simulink model "BLDCmotor_FOC_R2017b_fixdt_backup"  (R2017b)
settings: Solver=FixedStepDiscrete  StartTime=0  StopTime=0.5  FixedStep=Ts  MaxStep=1e-6  RelTol=1e-6  AbsTol=1e-6  EnableMultiTasking=on
PreLoadFcn:
  | addpath(pwd);
  | addpath(genpath('01_Libraries'));
  | addpath(genpath('02_Figures'));
  | addpath(genpath('03_CreateParamTable'));
InitFcn:
  | init_model;
values from neighbouring files (symbols this model uses):
  a_elecAngle = 60    [init_model.m]
  a_elecPeriod = 360    [init_model.m]
  a_phaAdvMax = 25    [init_model.m]
  b_angleMeasEna = 0    [init_model.m]
  b_cruiseCtrlEna = 0    [init_model.m]
  b_diagEna = 1    [init_model.m]
  b_fieldWeakEna = 0    [init_model.m]
  cf_currFilt = 0.12    [init_model.m]
  cf_idKi = 60 / (f_ctrl/3)    (= 0.01125)    [init_model.m]
  cf_idKp = 0.2    [init_model.m]
  cf_iqKi = 100 / (f_ctrl/3)    (= 0.01875)    [init_model.m]
  cf_iqKiLimProt = 60 / (f_ctrl/3)    (= 0.01125)    [init_model.m]
  cf_iqKp = 0.3    [init_model.m]
  cf_KbLimProt = 1000 / (f_ctrl/3)    (= 0.1875)    [init_model.m]
  cf_nKi = 20.4 / (f_ctrl/3)    (= 0.003825)    [init_model.m]
  cf_nKiLimProt = 20 / (f_ctrl/3)    (= 0.00375)    [init_model.m]
  cf_nKp = 1.18    [init_model.m]
  cf_speedCoef = round(f_ctrl * a_mechAngle * (pi/180) * (30/pi))    [init_model.m]
  CTRL_COM = 0    [init_model.m]
  CTRL_FOC = 2    [init_model.m]
  CTRL_SIN = 1    [init_model.m]
  dV_openRate = 1000 / (f_ctrl/3)    (= 0.1875)    [init_model.m]
  dz_cntTrnsDetHi = 40    [init_model.m]
  dz_cntTrnsDetLo = 20    [init_model.m]
  i_max = i_max * i_sca    (= 750)    [init_model.m]
  id_fieldWeakMax = 5 * i_sca    (= 250)    [init_model.m]
  iq_maxSca_M1 = sqrt(1 - iq_maxSca_XA.^2)    [init_model.m]
  n_commAcvLo = 15    [init_model.m]
  n_commDeacvHi = 30    [init_model.m]
  n_cruiseMotTgt = 0    [init_model.m]
  n_fieldWeakAuthHi = 400    [init_model.m]
  n_fieldWeakAuthLo = 300    [init_model.m]
  n_max = 1000    [init_model.m]
  n_polePairs = 15    [init_model.m]
  n_stdStillDet = 3    [init_model.m]
  OPEN_MODE = 0    [init_model.m]
  r_cos_M1 = cos((a_elecAngle_XA + 30)*(pi/180))    [init_model.m]
  r_errInpTgtThres = 600    [init_model.m]
  r_fieldWeakHi = 1000    [init_model.m]
  r_fieldWeakLo = 750    [init_model.m]
  r_sin3PhaA_M1 = sin3Arm + A*r_sinPhaA_M1    [init_model.m]
  r_sin3PhaB_M1 = sin3Arm + A*r_sinPhaB_M1    [init_model.m]
  r_sin3PhaC_M1 = sin3Arm + A*r_sinPhaC_M1    [init_model.m]
  r_sin_M1 = sin((a_elecAngle_XA + 30)*(pi/180))    [init_model.m]
  SPD_MODE = 2    [init_model.m]
  t_errDequal = 1.80 * f_ctrl/3    (= 9600)    [init_model.m]
  t_errQual = 0.24 * f_ctrl/3    (= 1280)    [init_model.m]
  TRQ_MODE = 3    [init_model.m]
  Ts = 5e-6    (= 5e-06)    [init_model.m]
  Ts_ctrl = 6e-5    (= 6e-05)    [init_model.m]
  Vd_max = 1000 - V_margin    (= 900)    [init_model.m]
  vec_hallToPos = [0 2 0 1 4 3 5 0]    [init_model.m]
  VLT_MODE = 1    [init_model.m]
  Vq_max_M1 = sqrt(Vd_max^2 - Vq_max_XA.^2)    [init_model.m]
  z_commutMap_M1 = [-1 -1  0  1  1  0 ... (first row only)    [init_model.m]
  z_ctrlModReq = VLT_MODE    (= 1)    [init_model.m]
  z_ctrlTypSel = CTRL_FOC    (= 2)    [init_model.m]
  z_maxCntRst = 2000    [init_model.m]
  z_selPhaCurMeasABC = 0    [init_model.m]
undefined symbols (not defined in the file or in its folder): DiscIntNeverNeededParam, sigbuilder_block
libraries: BLDC_controller_Lib x16, simulink x13, powerlib x6, pePwmGenerator x1
(part 3 of 4)

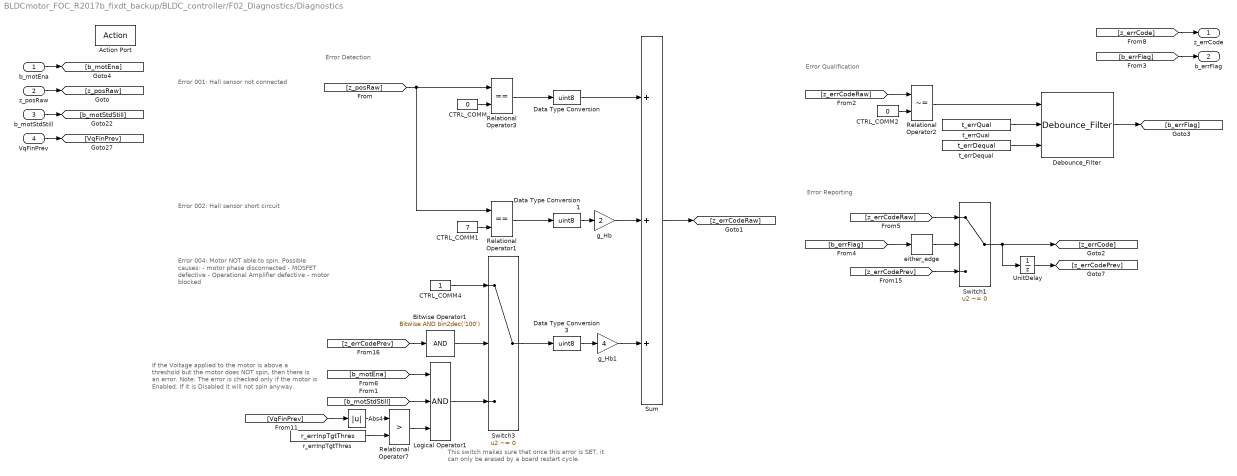
== system BLDCmotor_FOC_R2017b_fixdt_backup/BLDC_controller/F02_Diagnostics/Diagnostics ==
  note: Error 001: Hall sensor not connected
  note: Error 002: Hall sensor short circuit
  note: Error Qualification
  note: Error Detection
  note: Error Reporting
  note: Error 004: Motor NOT able to spin.
      |
      | Possible causes:
      | - motor phase disconnected
      | - MOSFET defective
      | - Operational Amplifier defective
      | - motor blocked
  note: This switch makes sure that once this error is SET, it can only be erased by a board restart cycle.
  note: If the Voltage applied to the motor is above a threshold but the motor does NOT spin, then there is an error.
      | Note: The error is checked only if the motor is Enabled. If it is Disabled it will not spin anyway.
  b_motEna : Inport
  z_posRaw : Inport  Port=2
  b_motStdStill : Inport  Port=3
  VqFinPrev : Inport  Port=4
  Action Port : ActionPort  ActionType=then
  Abs4 : Abs
  Bitwise Operator1 : simulink/Logic and Bit Operations/Bitwise Operator  logicop=AND  UseBitMask=on  BitMask=bin2dec('100')  BitMaskRealWorld=Stored Integer
  CTRL_COMM : Constant  Value=0  OutDataTypeStr=Inherit: Inherit via back propagation
  CTRL_COMM1 : Constant  Value=7  OutDataTypeStr=Inherit: Inherit via back propagation
  CTRL_COMM2 : Constant  Value=0  OutDataTypeStr=Inherit: Inherit via back propagation
  CTRL_COMM4 : Constant  OutDataTypeStr=Inherit: Inherit via back propagation
  Data Type Conversion : DataTypeConversion  OutDataTypeStr=uint8
  Data Type Conversion1 : DataTypeConversion  OutDataTypeStr=uint8
  Data Type Conversion3 : DataTypeConversion  OutDataTypeStr=uint8
  Debounce_Filter : BLDC_controller_Lib/Debounce_Filter
  Logical Operator1 : Logic  Inputs=3  AllPortsSameDT=off  OutDataTypeStr=boolean
  Relational Operator1 : RelationalOperator  Operator===  OutDataTypeStr=boolean  RndMeth=Simplest
  Relational Operator2 : RelationalOperator  Operator=~=  OutDataTypeStr=boolean  RndMeth=Simplest
  Relational Operator3 : RelationalOperator  Operator===  OutDataTypeStr=boolean  RndMeth=Simplest
  Relational Operator7 : RelationalOperator  Operator=>  OutDataTypeStr=boolean  RndMeth=Simplest
  Sum : Sum  Inputs=+++  RndMeth=Simplest  OutDataTypeStr=Inherit: Same as first input
  Switch1 : Switch  Criteria=u2 ~= 0  OutDataTypeStr=Inherit: Inherit via back propagation  RndMeth=Zero
  Switch3 : Switch  Criteria=u2 ~= 0  OutDataTypeStr=Inherit: Inherit via back propagation  RndMeth=Zero
  UnitDelay : UnitDelay  SampleTime=-1
      settings: AttributesFormatString=Ini=%<X0>
  either_edge : BLDC_controller_Lib/either_edge
  g_Hb : Gain  Gain=2  RndMeth=Simplest  OutDataTypeStr=Inherit: Same as input
  g_Hb1 : Gain  Gain=4  RndMeth=Simplest  OutDataTypeStr=Inherit: Same as input
  r_errInpTgtThres : Constant  Value=r_errInpTgtThres  OutDataTypeStr=Inherit: Inherit via back propagation
  t_errDequal : Constant  Value=t_errDequal  OutDataTypeStr=Inherit: Inherit via back propagation
  t_errQual : Constant  Value=t_errQual  OutDataTypeStr=Inherit: Inherit via back propagation
  "z_errCode " : Outport
  b_errFlag : Outport  Port=2
  wires:
  [z_errCode] -> "z_errCode "/1
  z_posRaw/1 -> [z_posRaw]
  t_errDequal/1 -> Debounce_Filter/3
  t_errQual/1 -> Debounce_Filter/2
  CTRL_COMM/1 -> Relational Operator3/2
  CTRL_COMM1/1 -> Relational Operator1/2
  [z_posRaw] -> Relational Operator1/1, Relational Operator3/1
  Relational Operator3/1 -> Data Type Conversion/1
  Sum/1 -> [z_errCodeRaw]
  Relational Operator2/1 -> Debounce_Filter/1
  [z_errCodeRaw] -> Relational Operator2/1
  CTRL_COMM2/1 -> Relational Operator2/2
  Debounce_Filter/1 -> [b_errFlag]
  either_edge/1 -> Switch1/2
  Switch1/1 -> [z_errCode], UnitDelay/1
  [b_errFlag] -> b_errFlag/1
  [b_errFlag] -> either_edge/1
  [z_errCodeRaw] -> Switch1/1
  g_Hb/1 -> Sum/2
  Relational Operator1/1 -> Data Type Conversion1/1
  Data Type Conversion/1 -> Sum/1
  Data Type Conversion1/1 -> g_Hb/1
  Switch3/1 -> Data Type Conversion3/1
  Data Type Conversion3/1 -> g_Hb1/1
  g_Hb1/1 -> Sum/3
  VqFinPrev/1 -> [VqFinPrev]
  b_motStdStill/1 -> [b_motStdStill]
  [VqFinPrev] -> Abs4/1
  Abs4/1 -> Relational Operator7/1
  r_errInpTgtThres/1 -> Relational Operator7/2
  UnitDelay/1 -> [z_errCodePrev]
  [z_errCodePrev] -> Switch1/3
  [z_errCodePrev] -> Bitwise Operator1/1
  Bitwise Operator1/1 -> Switch3/2
  CTRL_COMM4/1 -> Switch3/1
  Logical Operator1/1 -> Switch3/3
  b_motEna/1 -> [b_motEna]
  Relational Operator7/1 -> Logical Operator1/3
  [b_motEna] -> Logical Operator1/1
  [b_motStdStill] -> Logical Operator1/2

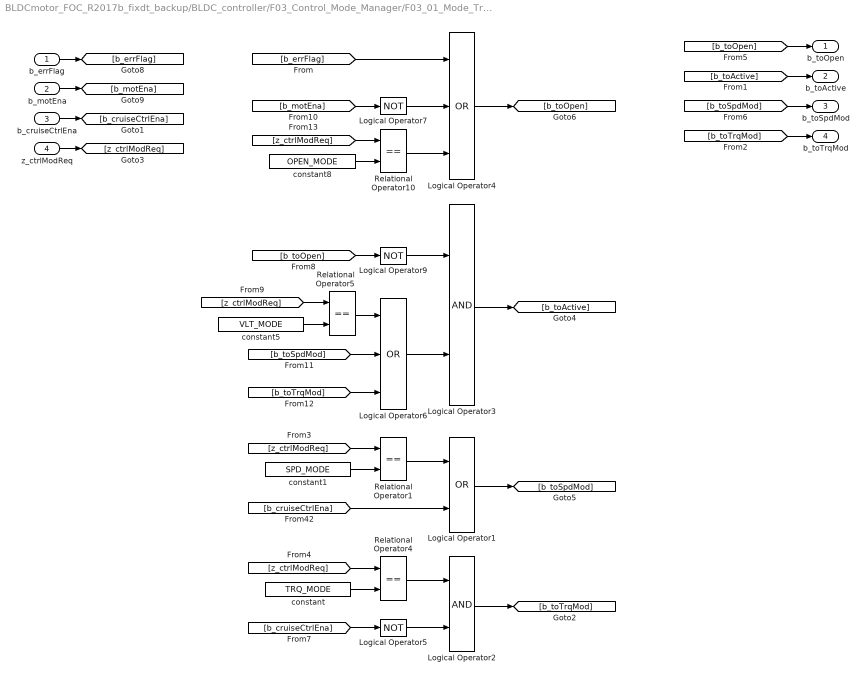
== system BLDCmotor_FOC_R2017b_fixdt_backup/BLDC_controller/F03_Control_Mode_Manager/F03_01_Mode_Transition_Calculation ==
  b_errFlag : Inport
  b_motEna : Inport  Port=2
  b_cruiseCtrlEna : Inport  Port=3
  z_ctrlModReq : Inport  Port=4
  Logical Operator1 : Logic  Operator=OR  AllPortsSameDT=off  OutDataTypeStr=boolean
  Logical Operator2 : Logic  AllPortsSameDT=off  OutDataTypeStr=boolean
  Logical Operator3 : Logic  AllPortsSameDT=off  OutDataTypeStr=boolean
  Logical Operator4 : Logic  Operator=OR  Inputs=3  AllPortsSameDT=off  OutDataTypeStr=boolean
  Logical Operator5 : Logic  Operator=NOT  AllPortsSameDT=off  OutDataTypeStr=boolean
  Logical Operator6 : Logic  Operator=OR  Inputs=3  AllPortsSameDT=off  OutDataTypeStr=boolean
  Logical Operator7 : Logic  Operator=NOT  AllPortsSameDT=off  OutDataTypeStr=boolean
  Logical Operator9 : Logic  Operator=NOT  AllPortsSameDT=off  OutDataTypeStr=boolean
  Relational Operator{1,4..5,10} (4 alike) : RelationalOperator  Operator===  OutDataTypeStr=boolean  RndMeth=Simplest
  constant : Constant  Value=TRQ_MODE  OutDataTypeStr=Inherit: Inherit via back propagation
  constant1 : Constant  Value=SPD_MODE  OutDataTypeStr=Inherit: Inherit via back propagation
  constant5 : Constant  Value=VLT_MODE  OutDataTypeStr=Inherit: Inherit via back propagation
  constant8 : Constant  Value=OPEN_MODE  OutDataTypeStr=Inherit: Inherit via back propagation
  b_toOpen : Outport  OutputWhenDisabled=reset  InitialOutput=0
  b_toActive : Outport  Port=2  OutputWhenDisabled=reset  InitialOutput=0
  b_toSpdMod : Outport  Port=3  OutputWhenDisabled=reset  InitialOutput=0
  b_toTrqMod : Outport  Port=4  OutputWhenDisabled=reset  InitialOutput=0
  wires:
  Logical Operator3/1 -> [b_toActive]
  [z_ctrlModReq] -> Relational Operator10/1
  constant5/1 -> Relational Operator5/2
  [z_ctrlModReq] -> Relational Operator4/1
  constant/1 -> Relational Operator4/2
  constant1/1 -> Relational Operator1/2
  [z_ctrlModReq] -> Relational Operator1/1
  Relational Operator5/1 -> Logical Operator6/1
  [z_ctrlModReq] -> Relational Operator5/1
  Logical Operator9/1 -> Logical Operator3/1
  Relational Operator10/1 -> Logical Operator4/3
  [b_motEna] -> Logical Operator7/1
  [b_toOpen] -> Logical Operator9/1
  Logical Operator4/1 -> [b_toOpen]
  constant8/1 -> Relational Operator10/2
  b_motEna/1 -> [b_motEna]
  z_ctrlModReq/1 -> [z_ctrlModReq]
  [b_toOpen] -> b_toOpen/1
  [b_toActive] -> b_toActive/1
  [b_toTrqMod] -> b_toTrqMod/1
  [b_toSpdMod] -> b_toSpdMod/1
  b_errFlag/1 -> [b_errFlag]
  [b_toSpdMod] -> Logical Operator6/2
  [b_toTrqMod] -> Logical Operator6/3
  Logical Operator6/1 -> Logical Operator3/2
  Relational Operator1/1 -> Logical Operator1/1
  Logical Operator1/1 -> [b_toSpdMod]
  [b_cruiseCtrlEna] -> Logical Operator1/2
  Relational Operator4/1 -> Logical Operator2/1
  Logical Operator2/1 -> [b_toTrqMod]
  [b_cruiseCtrlEna] -> Logical Operator5/1
  Logical Operator5/1 -> Logical Operator2/2
  Logical Operator7/1 -> Logical Operator4/2
  [b_errFlag] -> Logical Operator4/1
  b_cruiseCtrlEna/1 -> [b_cruiseCtrlEna]

== system BLDCmotor_FOC_R2017b_fixdt_backup/BLDC_controller/F03_Control_Mode_Manager/F03_03_Input_Target_Synthesis ==
  note: Input Scaling [-1000,1000] → [min,max]
  note: Final check if OPEN_MODE is requested
  z_ctrlTypSel : Inport
  z_ctrlModReq : Inport  Port=2
  z_ctrlMod : Inport  Port=3
  r_inpTgt : Inport  Port=4
  VqFinPrev : Inport  Port=5
  Default_Control_Type : Subsystem
  Default_Mode : Subsystem
  FOC_Control_Type : Subsystem
  If1 : If  IfExpression=u1 == CTRL_FOC
  If2 : If  IfExpression=u1 == OPEN_MODE
  Merge : Merge
  Merge1 : Merge
  Open_Mode : Subsystem
  Saturation : Saturate  UpperLimit=1000  LowerLimit=-1000
  r_inpTgtSca : Outport  OutputWhenDisabled=reset  InitialOutput=0
  wires:
  FOC_Control_Type/1(r_inpTgtScaFOC) -> Merge/1
  [r_inpTgt] -> FOC_Control_Type/1(r_inpTgt)
  [r_inpTgtSca] -> r_inpTgtSca/1
  If1/1 -> FOC_Control_Type/Action
  z_ctrlTypSel/1 -> [z_ctrlTypSel]
  [z_ctrlTypSel] -> If1/1
  Default_Control_Type/1(r_inpTgtScaDft) -> Merge/2
  [r_inpTgt] -> Default_Control_Type/1(r_inpTgt)
  r_inpTgt/1 -> Saturation/1
  Merge/1 -> [r_inpTgtScaRaw]
  If1/2 -> Default_Control_Type/Action
  [z_ctrlModReq] -> FOC_Control_Type/2(z_ctrlModReq)
  z_ctrlModReq/1 -> [z_ctrlModReq]
  z_ctrlMod/1 -> [z_ctrlMod]
  [z_ctrlMod] -> If2/1
  If2/1 -> Open_Mode/Action
  [VqFinPrev] -> Open_Mode/1(VqFinPrev)
  Open_Mode/1(r_inpTgtScaOpen) -> Merge1/1
  Default_Mode/1(r_inpTgtScaDft) -> Merge1/2
  Merge1/1 -> [r_inpTgtSca]
  [r_inpTgtScaRaw] -> Default_Mode/1(r_inpTgtScaRaw)
  If2/2 -> Default_Mode/Action
  VqFinPrev/1 -> [VqFinPrev]
  Saturation/1 -> [r_inpTgt]

== system BLDCmotor_FOC_R2017b_fixdt_backup/BLDC_controller/F04_Field_Weakening/Field_Weakening ==
  note: Calculate Blending Factor
  note: This blendig factor is a number between [0, 1]. It manages the Field weakening amount, ranging from 0 to a calibratable Max value.
  note: Field Weakening / Phase Advance
  z_ctrlTypSel : Inport
  r_inpTgt : Inport  Port=2
  n_motAbs : Inport  Port=3
  Action Port : ActionPort  ActionType=then
  Abs5 : Abs  OutDataTypeStr=Inherit: Inherit via back propagation  RndMeth=Zero
  CTRL_COMM2 : Constant  Value=CTRL_FOC  OutDataTypeStr=Inherit: Inherit via back propagation
  Divide1 : Product  Inputs=*/  OutDataTypeStr=fixdt(0,16,15)  RndMeth=Simplest
  Divide14 : Product  Inputs=*/  OutDataTypeStr=fixdt(0,16,15)  RndMeth=Simplest
  Divide2 : Product  Inputs=**  OutDataTypeStr=fixdt(0,16,15)  RndMeth=Simplest
  Divide3 : Product  Inputs=**  RndMeth=Simplest  OutDataTypeStr=Inherit: Same as first input
  Relational Operator1 : RelationalOperator  Operator===  OutDataTypeStr=boolean  RndMeth=Simplest
  Saturation Dynamic : simulink/Discontinuities/Saturation Dynamic  OutMin=[]  OutMax=[]  OutDataTypeStr=Inherit: Same as second input  OutDataType=fixdt(1, 16)  OutScaling=2^-10  DoSatur=off
  Saturation Dynamic1 : simulink/Discontinuities/Saturation Dynamic  OutMin=[]  OutMax=[]  OutDataTypeStr=Inherit: Same as second input  OutDataType=fixdt(1, 16)  OutScaling=2^-10  DoSatur=off
  Sum{1..4} (4 alike) : Sum  Inputs=+-  RndMeth=Simplest  OutDataTypeStr=Inherit: Same as first input
  Switch2 : Switch  Criteria=u2 ~= 0  OutDataTypeStr=Inherit: Inherit via back propagation  RndMeth=Zero
  a_phaAdvMax : Constant  Value=a_phaAdvMax  OutDataTypeStr=fixdt(1,16,4)
  id_fieldWeakMax : Constant  Value=id_fieldWeakMax  OutDataTypeStr=fixdt(1,16,4)
  n_fieldWeakAuthHi : Constant  Value=n_fieldWeakAuthHi  OutDataTypeStr=fixdt(1,16,4)
  n_fieldWeakAuthLo : Constant  Value=n_fieldWeakAuthLo  OutDataTypeStr=fixdt(1,16,4)
  r_fieldWeakHi : Constant  Value=r_fieldWeakHi  OutDataTypeStr=fixdt(1,16,4)
  r_fieldWeakLo : Constant  Value=r_fieldWeakLo  OutDataTypeStr=fixdt(1,16,4)
  "r_fieldWeak " : Outport
  wires:
  a_phaAdvMax/1 -> Switch2/3
  [r_fieldWeak] -> "r_fieldWeak "/1
  Switch2/1 -> Divide3/1
  n_fieldWeakAuthLo/1 -> Saturation Dynamic/3, Sum4/2, Sum2/2
  CTRL_COMM2/1 -> Relational Operator1/2
  Relational Operator1/1 -> Switch2/2
  [n_motAbs] -> Saturation Dynamic/2
  n_motAbs/1 -> [n_motAbs]
  Divide14/1 -> Divide2/1
  Saturation Dynamic/1 -> Sum4/1
  n_fieldWeakAuthHi/1 -> Saturation Dynamic/1, Sum2/1
  Divide1/1 -> Divide2/2
  Sum4/1 -> Divide1/1
  [r_blendFactor] -> Divide3/2
  Sum3/1 -> Divide14/2
  id_fieldWeakMax/1 -> Switch2/1
  [r_inpTgt] -> Abs5/1
  Saturation Dynamic1/1 -> Sum1/1
  Divide2/1 -> [r_blendFactor]
  Sum2/1 -> Divide1/2
  Abs5/1 -> Saturation Dynamic1/2
  z_ctrlTypSel/1 -> [z_ctrlTypSel]
  r_inpTgt/1 -> [r_inpTgt]
  r_fieldWeakHi/1 -> Saturation Dynamic1/1, Sum3/1
  r_fieldWeakLo/1 -> Saturation Dynamic1/3, Sum3/2, Sum1/2
  Divide3/1 -> [r_fieldWeak]
  Sum1/1 -> Divide14/1
  [z_ctrlTypSel] -> Relational Operator1/1

== system BLDCmotor_FOC_R2017b_fixdt_backup/BLDC_controller/F05_Field_Oriented_Control/Clarke_Transform ==
  i_phaAB : Inport
  i_phaBC : Inport  Port=2
  Clarke_PhasesAB : Subsystem
  Clarke_PhasesAC : Subsystem
  Clarke_PhasesBC : Subsystem
  If1 : If  IfExpression=u1 == 0  ElseIfExpressions=u1 == 1
  Merge1 : Merge  Inputs=3
  Merge2 : Merge  Inputs=3
  z_selPhaCurMeasABC : Constant  Value=z_selPhaCurMeasABC  OutDataTypeStr=uint8
  i_alpha : Outport
  i_beta : Outport  Port=2
  wires:
  Clarke_PhasesBC/1(i_alphaBC) -> [i_alphaBC]
  [i_betaBC] -> Merge1/2
  [i_betaAB] -> Merge1/1
  i_phaAB/1 -> [i_phaAB]
  [i_phaBC] -> Clarke_PhasesBC/2(i_phaC)
  [i_phaAB] -> Clarke_PhasesBC/1(i_phaB)
  Clarke_PhasesAB/1(i_alphaAB) -> [i_alphaAB]
  [i_alphaAB] -> Merge2/1
  If1/1 -> Clarke_PhasesAB/Action
  z_selPhaCurMeasABC/1 -> If1/1
  [i_alphaBC] -> Merge2/2
  [i_beta] -> i_beta/1
  Clarke_PhasesAB/2(i_betaAB) -> [i_betaAB]
  i_phaBC/1 -> [i_phaBC]
  [i_phaBC] -> Clarke_PhasesAB/2(i_phaB)
  Merge1/1 -> [i_beta]
  Merge2/1 -> [i_alpha]
  [i_phaAB] -> Clarke_PhasesAB/1(i_phaA)
  [i_alpha] -> i_alpha/1
  Clarke_PhasesBC/2(i_betaBC) -> [i_betaBC]
  If1/2 -> Clarke_PhasesBC/Action
  If1/3 -> Clarke_PhasesAC/Action
  [i_phaAB] -> Clarke_PhasesAC/1(i_phaA)
  [i_phaBC] -> Clarke_PhasesAC/2(i_phaC)
  Clarke_PhasesAC/2(i_betaAC) -> [i_betaAC]
  Clarke_PhasesAC/1(i_alphaAC) -> [i_alphaAC]
  [i_alphaAC] -> Merge2/3
  [i_betaAC] -> Merge1/3

== system BLDCmotor_FOC_R2017b_fixdt_backup/BLDC_controller/F05_Field_Oriented_Control/Current_Filtering ==
  iq_raw : Inport
  id_raw : Inport  Port=2
  Action Port : ActionPort  InitializeStates=reset  ActionType=then
  Abs5 : Abs  OutDataTypeStr=Inherit: Inherit via back propagation  RndMeth=Zero
  Demux1 : Demux  Outputs=2
  Low_Pass_Filter : BLDC_controller_Lib/Low_Pass_Filter  SystemSampleTime=-1
  Mux2 : Mux  Inputs=2
  cf_currFilt : Constant  Value=cf_currFilt  OutDataTypeStr=fixdt(0,16,16)
  iq : Outport  OutputWhenDisabled=reset  InitialOutput=0
  iqAbs : Outport  Port=2  OutputWhenDisabled=reset  InitialOutput=0
  id : Outport  Port=3  OutputWhenDisabled=reset  InitialOutput=0
  wires:
  Mux2/1 -> Low_Pass_Filter/1
  Demux1/2 -> [id]
  cf_currFilt/1 -> Low_Pass_Filter/2
  id_raw/1 -> [id_raw]
  [iq] -> Abs5/1, iq/1
  [id] -> id/1
  iq_raw/1 -> [iq_raw]
  Demux1/1 -> [iq]
  Low_Pass_Filter/1 -> Demux1/1
  [iq_raw] -> Mux2/1
  [id_raw] -> Mux2/2
  Abs5/1 -> iqAbs/1

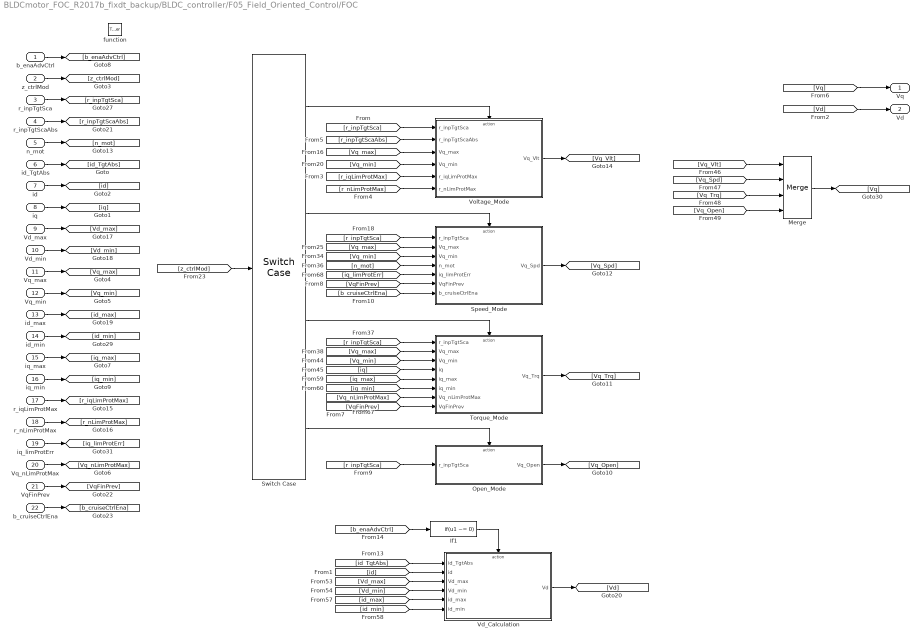
== system BLDCmotor_FOC_R2017b_fixdt_backup/BLDC_controller/F05_Field_Oriented_Control/FOC ==
  b_enaAdvCtrl : Inport
  z_ctrlMod : Inport  Port=2
  r_inpTgtSca : Inport  Port=3
  r_inpTgtScaAbs : Inport  Port=4
  n_mot : Inport  Port=5
  id_TgtAbs : Inport  Port=6
  id : Inport  Port=7
  iq : Inport  Port=8
  Vd_max : Inport  Port=9
  Vd_min : Inport  Port=10
  Vq_max : Inport  Port=11
  Vq_min : Inport  Port=12
  id_max : Inport  Port=13
  id_min : Inport  Port=14
  iq_max : Inport  Port=15
  iq_min : Inport  Port=16
  r_iqLimProtMax : Inport  Port=17
  r_nLimProtMax : Inport  Port=18
  iq_limProtErr : Inport  Port=19
  Vq_nLimProtMax : Inport  Port=20
  VqFinPrev : Inport  Port=21
  b_cruiseCtrlEna : Inport  Port=22
  function : TriggerPort  TriggerType=function-call  VariantControl=Variant
  If1 : If  IfExpression=u1 ~= 0  ShowElse=off
  Merge : Merge  Inputs=4
  Open_Mode : Subsystem
  Speed_Mode : Subsystem
  Switch Case : SwitchCase  CaseConditions={VLT_MODE, SPD_MODE, TRQ_MODE}
  Torque_Mode : Subsystem
  Vd_Calculation : Subsystem
  Voltage_Mode : Subsystem
  Vq : Outport
  Vd : Outport  Port=2
  wires:
  [id_TgtAbs] -> Vd_Calculation/1(id_TgtAbs)
  [z_ctrlMod] -> Switch Case/1
  If1/1 -> Vd_Calculation/Action
  [id] -> Vd_Calculation/2(id)
  [b_enaAdvCtrl] -> If1/1
  Torque_Mode/1(Vq_Trq) -> [Vq_Trq]
  [Vq_max] -> Torque_Mode/2(Vq_max)
  [r_inpTgtSca] -> Torque_Mode/1(r_inpTgtSca)
  [iq] -> Torque_Mode/4(iq)
  Switch Case/3 -> Torque_Mode/Action
  [Vq_min] -> Speed_Mode/3(Vq_min)
  [Vq_Vlt] -> Merge/1
  [n_mot] -> Speed_Mode/4(n_mot)
  [Vq_max] -> Speed_Mode/2(Vq_max)
  Switch Case/2 -> Speed_Mode/Action
  [Vq_Open] -> Merge/4
  [r_inpTgtSca] -> Voltage_Mode/1(r_inpTgtSca)
  [r_inpTgtSca] -> Speed_Mode/1(r_inpTgtSca)
  [Vq_min] -> Torque_Mode/3(Vq_min)
  [Vq_max] -> Voltage_Mode/3(Vq_max)
  [Vq_min] -> Voltage_Mode/4(Vq_min)
  Switch Case/1 -> Voltage_Mode/Action
  Switch Case/4 -> Open_Mode/Action
  [Vq_Spd] -> Merge/2
  [Vq_Trq] -> Merge/3
  Speed_Mode/1(Vq_Spd) -> [Vq_Spd]
  Open_Mode/1(Vq_Open) -> [Vq_Open]
  Voltage_Mode/1(Vq_Vlt) -> [Vq_Vlt]
  [Vd_max] -> Vd_Calculation/3(Vd_max)
  [iq_max] -> Torque_Mode/5(iq_max)
  [r_inpTgtSca] -> Open_Mode/1(r_inpTgtSca)
  [id_min] -> Vd_Calculation/6(id_min)
  [id_max] -> Vd_Calculation/5(id_max)
  [iq_min] -> Torque_Mode/6(iq_min)
  [Vq_nLimProtMax] -> Torque_Mode/7(Vq_nLimProtMax)
  [Vd_min] -> Vd_Calculation/4(Vd_min)
  [iq_limProtErr] -> Speed_Mode/5(iq_limProtErr)
  [Vq] -> Vq/1
  [Vd] -> Vd/1
  r_inpTgtSca/1 -> [r_inpTgtSca]
  z_ctrlMod/1 -> [z_ctrlMod]
  b_enaAdvCtrl/1 -> [b_enaAdvCtrl]
  iq/1 -> [iq]
  id_min/1 -> [id_min]
  id_max/1 -> [id_max]
  Vd_max/1 -> [Vd_max]
  id_TgtAbs/1 -> [id_TgtAbs]
  id/1 -> [id]
  Vd_min/1 -> [Vd_min]
  Vq_min/1 -> [Vq_min]
  Vq_max/1 -> [Vq_max]
  Vq_nLimProtMax/1 -> [Vq_nLimProtMax]
  iq_limProtErr/1 -> [iq_limProtErr]
  iq_min/1 -> [iq_min]
  iq_max/1 -> [iq_max]
  n_mot/1 -> [n_mot]
  r_iqLimProtMax/1 -> [r_iqLimProtMax]
  r_nLimProtMax/1 -> [r_nLimProtMax]
  [r_iqLimProtMax] -> Voltage_Mode/5(r_iqLimProtMax)
  [r_nLimProtMax] -> Voltage_Mode/6(r_nLimProtMax)
  r_inpTgtScaAbs/1 -> [r_inpTgtScaAbs]
  [r_inpTgtScaAbs] -> Voltage_Mode/2(r_inpTgtScaAbs)
  VqFinPrev/1 -> [VqFinPrev]
  [VqFinPrev] -> Torque_Mode/8(VqFinPrev)
  [VqFinPrev] -> Speed_Mode/6(VqFinPrev)
  [b_cruiseCtrlEna] -> Speed_Mode/7(b_cruiseCtrlEna)
  b_cruiseCtrlEna/1 -> [b_cruiseCtrlEna]
  Vd_Calculation/1(Vd) -> [Vd]
  Merge/1 -> [Vq]

== system BLDCmotor_FOC_R2017b_fixdt_backup/BLDC_controller/F05_Field_Oriented_Control/Inv_Clarke_Transform ==
  note: Inverse Clarke Transform:
      | V_phaA = V_alpha
      | V_phaB = -(1/2)*V_alpha + (sqrt(3)/2)*V_beta
      | V_phaC = -VphaA - V_phaB
  note: Space Vector Modulation (SVM)
  V_alpha : Inport
  V_beta : Inport  Port=2
  Add : Sum  SaturateOnIntegerOverflow=on
  Add1 : Sum  Inputs=-+  SaturateOnIntegerOverflow=on  OutDataTypeStr=Inherit: Same as first input
  Gain1 : Gain  Tag=struct('comment',struct('text','','placement',1),'logdata',struct('maxnumvals',inf,'plotchannels',[],'loggingmode',3,'channels',1),'output',struct('variable','','description','','name','$S_$B','width',1,'address','','max',NaN,'min',NaN,'class','default','type','CONTINUOUS','scaling','','lsb',1,'offset',0,'arb',0,'freeze',1,'unit','','autoscalingmode',1,'lowerheadroom',1,'upperheadroom',1,'headroomunit','bit','keepdatatype',1,'checkmin',0,'checkmax',0,'castoutput',0,'show',0),'gain',struct('variable','','description','','name','$S_$B_gain','width',1,'address','','max',NaN,'min',NaN,'class','default','type','CONTINUOUS','scaling','','lsb',1,'offset',0,'arb',0,'freeze',1,'unit','','keepdatatype',1,'value','1','scalar',0,'tolerance',1),'scalingvalid',0,'date',730486)  Gain=sqrt(3)/2  RndMeth=Zero  OutDataTypeStr=Inherit: Same as input
  Gain2 : Gain  Gain=0.5  OutDataTypeStr=Inherit: Same as input
  Gain3 : Gain  Tag=struct('comment',struct('text','','placement',1),'logdata',struct('maxnumvals',inf,'plotchannels',[],'loggingmode',3,'channels',1),'output',struct('variable','','description','','name','$S_$B','width',1,'address','','max',NaN,'min',NaN,'class','default','type','CONTINUOUS','scaling','','lsb',1,'offset',0,'arb',0,'freeze',1,'unit','','autoscalingmode',1,'lowerheadroom',1,'upperheadroom',1,'headroomunit','bit','keepdatatype',1,'checkmin',0,'checkmax',0,'castoutput',0,'show',0),'gain',struct('variable','','description','','name','$S_$B_gain','width',1,'address','','max',NaN,'min',NaN,'class','default','type','CONTINUOUS','scaling','','lsb',1,'offset',0,'arb',0,'freeze',1,'unit','','keepdatatype',1,'value','1','scalar',0,'tolerance',1),'scalingvalid',0,'date',730486)  Gain=1/2  RndMeth=Zero  OutDataTypeStr=Inherit: Same as input
  Gain4 : Gain  Gain=2/sqrt(3)  OutDataTypeStr=Inherit: Same as input
  MinMax1 : MinMax  InputSameDT=on
  MinMax2 : MinMax  Function=max  InputSameDT=on
  Mux4 : Mux  Inputs=3
  Sum2 : Sum  Inputs=--  RndMeth=Simplest  SaturateOnIntegerOverflow=on  OutDataTypeStr=Inherit: Same as first input
  Sum6 : Sum  Inputs=-+  RndMeth=Simplest  SaturateOnIntegerOverflow=on  OutDataTypeStr=Inherit: Same as first input
  V_phaABC_FOC : Outport
  wires:
  Sum6/1 -> Sum2/2, Mux4/2
  Sum2/1 -> Mux4/3
  Gain1/1 -> Sum6/2
  Gain3/1 -> Sum6/1
  V_alpha/1 -> Gain3/1, Sum2/1, Mux4/1  "alpha"
  V_beta/1 -> Gain1/1  "beta"
  Add/1 -> Gain2/1
  Add1/1 -> Gain4/1
  MinMax1/1 -> Add/1
  Gain2/1 -> Add1/1
  Gain4/1 -> V_phaABC_FOC/1
  MinMax2/1 -> Add/2
  Mux4/1 -> Add1/2, MinMax2/1, MinMax1/1

== system BLDCmotor_FOC_R2017b_fixdt_backup/BLDC_controller/F05_Field_Oriented_Control/Inv_Park_Transform ==
  note: Inverse Park Transform:
      | V_alpha = Vd*cos(angle) - Vq*sin(angle)
      | V_beta = Vd*sin(angle) + Vq*cos(angle)
  Vq : Inport
  Vd : Inport  Port=2
  r_sin : Inport  Port=3
  r_cos : Inport  Port=4
  Divide{1..4} (4 alike) : Product  Inputs=**  RndMeth=Simplest  OutDataTypeStr=Inherit: Same as first input
  Sum1 : Sum  RndMeth=Simplest  SaturateOnIntegerOverflow=on  OutDataTypeStr=Inherit: Same as first input
  Sum6 : Sum  Inputs=+-  RndMeth=Simplest  SaturateOnIntegerOverflow=on  OutDataTypeStr=Inherit: Same as first input
  V_alpha : Outport
  V_beta : Outport  Port=2
  wires:
  r_sin/1 -> [r_sin]
  Vd/1 -> [Vd]
  Vq/1 -> [Vq]
  r_cos/1 -> [r_cos]
  [r_cos] -> Divide4/2
  [r_sin] -> Divide1/2
  [Vd] -> Divide4/1
  [r_cos] -> Divide3/2
  Divide1/1 -> Sum6/2
  [Vq] -> Divide1/1
  [Vd] -> Divide2/1
  Divide2/1 -> Sum1/1
  Divide3/1 -> Sum1/2
  [Vq] -> Divide3/1
  Divide4/1 -> Sum6/1
  [r_sin] -> Divide2/2
  Sum1/1 -> V_beta/1
  Sum6/1 -> V_alpha/1

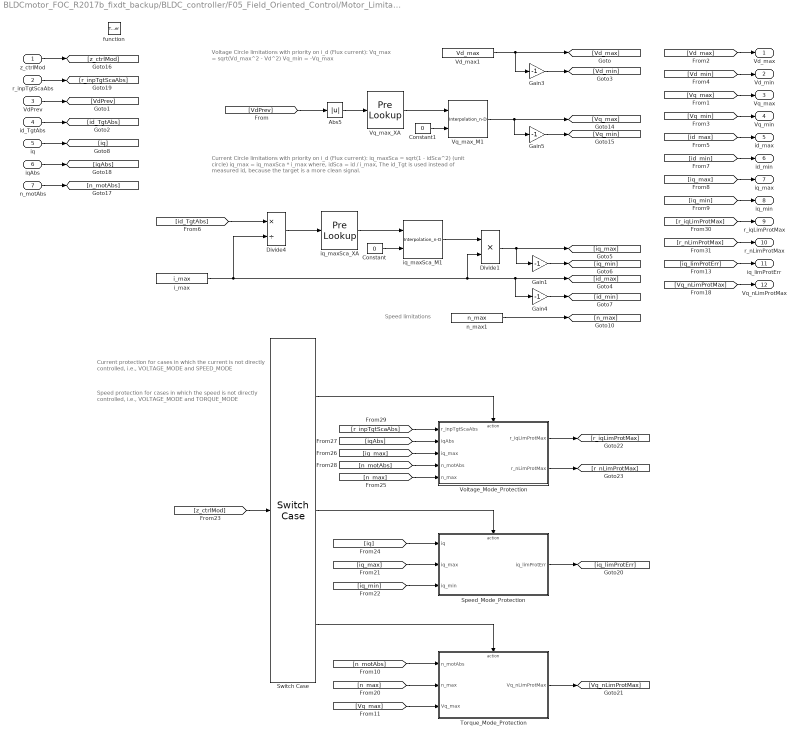
== system BLDCmotor_FOC_R2017b_fixdt_backup/BLDC_controller/F05_Field_Oriented_Control/Motor_Limitations ==
  note: Voltage Circle limitations with priority on i_d (Flux current):
      | Vq_max = sqrt(Vd_max^2 - Vd^2)
      | Vq_min = -Vq_max
  note: Current Circle limitations with priority on i_d (Flux current):
      | iq_maxSca = sqrt(1 - idSca^2) (unit circle)
      | iq_max = iq_maxSca * i_max
      |
      | where, idSca = id / i_max,
      |
      | The id_Tgt is used instead of measured id, because the target is a more clean signal.
  note: Speed limitations
  note: Current protection
      | for cases in which the current is not directly controlled, i.e., VOLTAGE_MODE and SPEED_MODE
  note: Speed protection
      | for cases in which the speed is not directly controlled, i.e., VOLTAGE_MODE and TORQUE_MODE
  z_ctrlMod : Inport
  r_inpTgtScaAbs : Inport  Port=2
  VdPrev : Inport  Port=3
  id_TgtAbs : Inport  Port=4
  iq : Inport  Port=5
  iqAbs : Inport  Port=6
  n_motAbs : Inport  Port=7
  function : TriggerPort  TriggerType=function-call  VariantControl=Variant
  Abs5 : Abs  OutDataTypeStr=Inherit: Inherit via back propagation  RndMeth=Zero
  Constant : Constant  Value=0  OutDataTypeStr=uint8
  Constant1 : Constant  Value=0  OutDataTypeStr=uint8
  Divide1 : Product  Inputs=**  OutDataTypeStr=fixdt(1,16,4)  RndMeth=Simplest
  Divide4 : Product  Inputs=*/  OutDataTypeStr=fixdt(0,16,16)  RndMeth=Simplest  SaturateOnIntegerOverflow=on
  Gain{1,3..5} (4 alike) : Gain  Tag=struct('comment',struct('text','','placement',1),'logdata',struct('maxnumvals',inf,'plotchannels',[],'loggingmode',3,'channels',1),'output',struct('variable','','description','','name','$S_$B','width',1,'address','','max',NaN,'min',NaN,'class','default','type','CONTINUOUS','scaling','','lsb',1,'offset',0,'arb',0,'freeze',1,'unit','','autoscalingmode',1,'lowerheadroom',1,'upperheadroom',1,'headroomunit','bit','keepdatatype',1,'checkmin',0,'checkmax',0,'castoutput',0,'show',0),'gain',struct('variable','','description','','name','$S_$B_gain','width',1,'address','','max',NaN,'min',NaN,'class','default','type','CONTINUOUS','scaling','','lsb',1,'offset',0,'arb',0,'freeze',1,'unit','','keepdatatype',1,'value','1','scalar',0,'tolerance',1),'scalingvalid',0,'date',730486)  Gain=-1  RndMeth=Zero  OutDataTypeStr=Inherit: Same as input  ParamDataTypeStr=Inherit: Same as input
  Speed_Mode_Protection : Subsystem
  Switch Case : SwitchCase  CaseConditions={VLT_MODE, SPD_MODE, TRQ_MODE}  ShowDefaultCase=off
  Torque_Mode_Protection : Subsystem
  Vd_max1 : Constant  Value=Vd_max  OutDataTypeStr=fixdt(1,16,4)
  Voltage_Mode_Protection : Subsystem
  Vq_max_M1 : Interpolation_n-D  NumberOfTableDimensions=1  Table=Vq_max_M1  InterpMethod=Flat  ExtrapMethod=Clip  DiagnosticForOutOfRangeInput=Error  RemoveProtectionIndex=on  ValidIndexMayReachLast=on  OutDataTypeStr=fixdt(1,16,4)  InternalRulePriority=Speed  RndMeth=Simplest
      settings: InputPortMap=u0,u1
  Vq_max_XA : PreLookup  BreakpointsData=Vq_max_XA  OutputSelection=Index only  IndexSearchMethod=Evenly spaced points  BeginIndexSearchUsingPreviousIndexResult=on  IndexDataTypeStr=uint8  FractionDataTypeStr=fixdt(0,8,6)  RndMeth=Simplest
  i_max : Constant  Value=i_max  OutDataTypeStr=fixdt(1,16,4)
  iq_maxSca_M1 : Interpolation_n-D  NumberOfTableDimensions=1  Table=iq_maxSca_M1  InterpMethod=Flat  ExtrapMethod=Clip  DiagnosticForOutOfRangeInput=Error  RemoveProtectionIndex=on  ValidIndexMayReachLast=on  OutDataTypeStr=fixdt(0,16,16)  InternalRulePriority=Speed  RndMeth=Simplest
      settings: InputPortMap=u0,u1
  iq_maxSca_XA : PreLookup  BreakpointsData=iq_maxSca_XA  OutputSelection=Index only  IndexSearchMethod=Evenly spaced points  BeginIndexSearchUsingPreviousIndexResult=on  IndexDataTypeStr=uint8  FractionDataTypeStr=fixdt(0,8,6)  RndMeth=Simplest
  n_max1 : Constant  Value=n_max  OutDataTypeStr=fixdt(1,16,4)
  Vd_max : Outport  InitialOutput=900
  Vd_min : Outport  Port=2  InitialOutput=-900
  Vq_max : Outport  Port=3  InitialOutput=900
  Vq_min : Outport  Port=4  InitialOutput=-900
  id_max : Outport  Port=5  InitialOutput=750
  id_min : Outport  Port=6  InitialOutput=-750
  iq_max : Outport  Port=7  InitialOutput=750
  iq_min : Outport  Port=8  InitialOutput=-750
  r_iqLimProtMax : Outport  Port=9
  r_nLimProtMax : Outport  Port=10
  iq_limProtErr : Outport  Port=11
  Vq_nLimProtMax : Outport  Port=12
  wires:
  Vq_max_XA/1 -> Vq_max_M1/1
  [Vq_min] -> Vq_min/1
  [Vq_max] -> Vq_max/1
  Gain5/1 -> [Vq_min]
  Vd_max1/1 -> Gain3/1, [Vd_max]
  [VdPrev] -> Abs5/1
  VdPrev/1 -> [VdPrev]
  id_TgtAbs/1 -> [id_TgtAbs]
  [Vd_max] -> Vd_max/1
  [Vd_min] -> Vd_min/1
  Gain3/1 -> [Vd_min]
  Gain4/1 -> [id_min]
  i_max/1 -> Divide1/2, [id_max], Gain4/1, Divide4/2
  Divide4/1 -> iq_maxSca_XA/1
  Divide1/1 -> [iq_max], Gain1/1
  Gain1/1 -> [iq_min]
  iq_maxSca_XA/1 -> iq_maxSca_M1/1
  [id_min] -> id_min/1
  [id_max] -> id_max/1
  [iq_max] -> iq_max/1
  [iq_min] -> iq_min/1
  iq/1 -> [iq]
  [iq_limProtErr] -> iq_limProtErr/1
  n_max1/1 -> [n_max]
  [Vq_nLimProtMax] -> Vq_nLimProtMax/1
  z_ctrlMod/1 -> [z_ctrlMod]
  Constant/1 -> iq_maxSca_M1/2
  Vq_max_M1/1 -> Gain5/1, [Vq_max]
  Constant1/1 -> Vq_max_M1/2
  Abs5/1 -> Vq_max_XA/1
  [id_TgtAbs] -> Divide4/1
  iq_maxSca_M1/1 -> Divide1/1
  [z_ctrlMod] -> Switch Case/1
  Switch Case/1 -> Voltage_Mode_Protection/Action
  Switch Case/2 -> Speed_Mode_Protection/Action
  Switch Case/3 -> Torque_Mode_Protection/Action
  [n_max] -> Torque_Mode_Protection/2(n_max)
  [iq] -> Speed_Mode_Protection/1(iq)
  [iq_min] -> Speed_Mode_Protection/3(iq_min)
  [iq_max] -> Speed_Mode_Protection/2(iq_max)
  [n_max] -> Voltage_Mode_Protection/5(n_max)
  [iq_max] -> Voltage_Mode_Protection/3(iq_max)
  n_motAbs/1 -> [n_motAbs]
  iqAbs/1 -> [iqAbs]
  [iqAbs] -> Voltage_Mode_Protection/2(iqAbs)
  [n_motAbs] -> Voltage_Mode_Protection/4(n_motAbs)
  r_inpTgtScaAbs/1 -> [r_inpTgtScaAbs]
  [r_inpTgtScaAbs] -> Voltage_Mode_Protection/1(r_inpTgtScaAbs)
  [r_nLimProtMax] -> r_nLimProtMax/1
  [r_iqLimProtMax] -> r_iqLimProtMax/1
  Speed_Mode_Protection/1(iq_limProtErr) -> [iq_limProtErr]
  Torque_Mode_Protection/1(Vq_nLimProtMax) -> [Vq_nLimProtMax]
  Voltage_Mode_Protection/1(r_iqLimProtMax) -> [r_iqLimProtMax]
  Voltage_Mode_Protection/2(r_nLimProtMax) -> [r_nLimProtMax]
  [n_motAbs] -> Torque_Mode_Protection/1(n_motAbs)
  [Vq_max] -> Torque_Mode_Protection/3(Vq_max)

== system BLDCmotor_FOC_R2017b_fixdt_backup/BLDC_controller/F05_Field_Oriented_Control/Park_Transform ==
  note: Park Transform:
      | iq = -i_alpha*sin(angle) + i_beta*cos(angle)
      | id = i_alpha*cos(angle) + i_beta*sin(angle)
  i_apha : Inport
  i_beta : Inport  Port=2
  r_sin : Inport  Port=3
  r_cos : Inport  Port=4
  Divide{1..4} (4 alike) : Product  Inputs=**  RndMeth=Simplest  OutDataTypeStr=Inherit: Same as first input
  Sum1 : Sum  OutDataTypeStr=fixdt(1,16,4)  RndMeth=Simplest  SaturateOnIntegerOverflow=on
  Sum6 : Sum  Inputs=-+  OutDataTypeStr=fixdt(1,16,4)  RndMeth=Simplest  SaturateOnIntegerOverflow=on
  iq_Raw : Outport
  id_Raw : Outport  Port=2
  wires:
  r_sin/1 -> [r_sin]
  i_beta/1 -> [i_beta]
  i_apha/1 -> [i_apha]
  r_cos/1 -> [r_cos]
  [r_sin] -> Divide4/2
  [i_apha] -> Divide4/1
  Divide4/1 -> Sum6/1
  Divide1/1 -> Sum6/2
  [i_beta] -> Divide1/1
  [r_cos] -> Divide1/2
  Sum6/1 -> iq_Raw/1
  Divide2/1 -> Sum1/1
  [i_apha] -> Divide2/1
  [r_cos] -> Divide2/2
  Divide3/1 -> Sum1/2
  [i_beta] -> Divide3/1
  [r_sin] -> Divide3/2
  Sum1/1 -> id_Raw/1

== system BLDCmotor_FOC_R2017b_fixdt_backup/BLDC_controller/F05_Field_Oriented_Control/Sine_Cosine_Approximation ==
  note: Sine/Cosine Look-up Tables
  note: Note: The Sine and Cosine maps are shifted in phase by 30 deg to align with the Hall sensors position.
  a_elecAngle : Inport
  Constant : Constant  Value=0  OutDataTypeStr=uint8
  a_elecAngle_XA : PreLookup  BreakpointsData=a_elecAngle_XA  OutputSelection=Index only  IndexSearchMethod=Evenly spaced points  BeginIndexSearchUsingPreviousIndexResult=on  IndexDataTypeStr=uint8  FractionDataTypeStr=fixdt(0,16,14)  RndMeth=Simplest
  r_cos_M1 : Interpolation_n-D  NumberOfTableDimensions=1  Table=r_cos_M1  InterpMethod=Flat  ExtrapMethod=Clip  DiagnosticForOutOfRangeInput=Error  RemoveProtectionIndex=on  ValidIndexMayReachLast=on  OutDataTypeStr=fixdt(1,16,14)  InternalRulePriority=Speed  RndMeth=Simplest
      settings: InputPortMap=u0,u1
  r_sin_M1 : Interpolation_n-D  NumberOfTableDimensions=1  Table=r_sin_M1  InterpMethod=Flat  ExtrapMethod=Clip  DiagnosticForOutOfRangeInput=Error  RemoveProtectionIndex=on  ValidIndexMayReachLast=on  OutDataTypeStr=fixdt(1,16,14)  InternalRulePriority=Speed  RndMeth=Simplest
      settings: InputPortMap=u0,u1
  r_sin : Outport
  r_cos : Outport  Port=2
  wires:
  a_elecAngle_XA/1 -> r_cos_M1/1, r_sin_M1/1
  [a_elecAngle] -> a_elecAngle_XA/1
  Constant/1 -> r_cos_M1/2, r_sin_M1/2
  a_elecAngle/1 -> [a_elecAngle]
  [r_sin] -> r_sin/1
  r_sin_M1/1 -> [r_sin]
  [r_cos] -> r_cos/1
  r_cos_M1/1 -> [r_cos]

== system BLDCmotor_FOC_R2017b_fixdt_backup/BLDC_controller/F06_Control_Type_Management/COM_Method ==
  VqFin : Inport
  z_pos : Inport  Port=2
  Action Port : ActionPort  ActionType=else
  Divide2 : Product  Inputs=**  RndMeth=Simplest  OutDataTypeStr=Inherit: Same as first input
  z_commutMap_M1 : LookupNDDirect  InputsSelectThisObjectFromTable=Column  Table=z_commutMap_M1  DiagnosticForOutOfRangeInput=None  TableDataTypeStr=int8
  V_phaABC_COM : Outport
  wires:
  Divide2/1 -> [V_phaABC_COM]
  [z_pos] -> z_commutMap_M1/1
  z_commutMap_M1/1 -> Divide2/2
  [VqFin] -> Divide2/1
  VqFin/1 -> [VqFin]
  z_pos/1 -> [z_pos]
  [V_phaABC_COM] -> V_phaABC_COM/1

== system BLDCmotor_FOC_R2017b_fixdt_backup/BLDC_controller/F06_Control_Type_Management/FOC_Method ==
  V_phaABC_FOC_in : Inport
  Action Port : ActionPort  ActionType=then
  V_phaABC_FOC : Outport
  wires:
  V_phaABC_FOC_in/1 -> V_phaABC_FOC/1

== system BLDCmotor_FOC_R2017b_fixdt_backup/BLDC_controller/F06_Control_Type_Management/SIN_Method ==
  note: Sinusoidal With 3rd Harmonic
  VqFin : Inport
  a_elecAngle : Inport  Port=2
  z_dir : Inport  Port=3
  r_fieldWeak : Inport  Port=4
  Action Port : ActionPort  ActionType=elseif
  Constant : Constant  Value=0  OutDataTypeStr=uint8
  Divide2 : Product  Inputs=**  RndMeth=Simplest  OutDataTypeStr=Inherit: Same as first input
  Final_Phase_Advance_Calculation : Subsystem
  Mux2 : Mux  Inputs=3
  a_elecAngle_XA : PreLookup  BreakpointsData=a_elecAngle_XA  OutputSelection=Index only  IndexSearchMethod=Evenly spaced points  BeginIndexSearchUsingPreviousIndexResult=on  IndexDataTypeStr=uint8  RndMeth=Simplest
  r_sin3PhaA_M1 : Interpolation_n-D  NumberOfTableDimensions=1  Table=r_sin3PhaA_M1  InterpMethod=Flat  ExtrapMethod=Clip  RemoveProtectionIndex=on  ValidIndexMayReachLast=on  OutDataTypeStr=fixdt(1,16,14)  InternalRulePriority=Speed  RndMeth=Simplest
      settings: InputPortMap=u0,u1
  r_sin3PhaB_M1 : Interpolation_n-D  NumberOfTableDimensions=1  Table=r_sin3PhaB_M1  InterpMethod=Flat  ExtrapMethod=Clip  RemoveProtectionIndex=on  ValidIndexMayReachLast=on  OutDataTypeStr=fixdt(1,16,14)  InternalRulePriority=Speed  RndMeth=Simplest
      settings: InputPortMap=u0,u1
  r_sin3PhaC_M1 : Interpolation_n-D  NumberOfTableDimensions=1  Table=r_sin3PhaC_M1  InterpMethod=Flat  ExtrapMethod=Clip  RemoveProtectionIndex=on  ValidIndexMayReachLast=on  OutDataTypeStr=fixdt(1,16,14)  InternalRulePriority=Speed  RndMeth=Simplest
      settings: InputPortMap=u0,u1
  V_phaABC_SIN : Outport
  wires:
  a_elecAngle_XA/1 -> r_sin3PhaC_M1/1, r_sin3PhaB_M1/1, r_sin3PhaA_M1/1
  Constant/1 -> r_sin3PhaC_M1/2, r_sin3PhaB_M1/2, r_sin3PhaA_M1/2
  Final_Phase_Advance_Calculation/1(a_elecAngleAdv) -> a_elecAngle_XA/1
  a_elecAngle/1 -> [a_elecAngle]
  r_fieldWeak/1 -> [r_fieldWeak]
  z_dir/1 -> [z_dir]
  VqFin/1 -> [VqFin]
  [a_elecAngle] -> Final_Phase_Advance_Calculation/1(a_elecAngle)
  [z_dir] -> Final_Phase_Advance_Calculation/2(z_dir)
  [r_fieldWeak] -> Final_Phase_Advance_Calculation/3(r_fieldWeak)
  [V_phaABC_SIN] -> V_phaABC_SIN/1
  [VqFin] -> Divide2/1
  r_sin3PhaA_M1/1 -> Mux2/1
  r_sin3PhaB_M1/1 -> Mux2/2
  r_sin3PhaC_M1/1 -> Mux2/3
  Mux2/1 -> Divide2/2
  Divide2/1 -> [V_phaABC_SIN]

== system BLDCmotor_FOC_R2017b_fixdt_backup/PWM_gates/PWM_generator1/__InputSSForSFun__ ==
  DC : Inport  SampleTime=Ts
  __UniqueOutportName__1__ : Outport
  wires:
  DC/1 -> __UniqueOutportName__1__/1

== system BLDCmotor_FOC_R2017b_fixdt_backup/PWM_gates/PWM_generator1/__OutputSSForSFun__ ==
  __UniqueInportName__1__ : Inport
  PWM : Outport
  wires:
  __UniqueInportName__1__/1 -> PWM/1

== system BLDCmotor_FOC_R2017b_fixdt_backup/PWM_gates/PWM_generator12/__InputSSForSFun__ ==
  DC : Inport  SampleTime=Ts
  __UniqueOutportName__1__ : Outport
  wires:
  DC/1 -> __UniqueOutportName__1__/1

== system BLDCmotor_FOC_R2017b_fixdt_backup/PWM_gates/PWM_generator12/__OutputSSForSFun__ ==
  __UniqueInportName__1__ : Inport
  PWM : Outport
  wires:
  __UniqueInportName__1__/1 -> PWM/1

== system BLDCmotor_FOC_R2017b_fixdt_backup/PWM_gates/PWM_generator2/__InputSSForSFun__ ==
  DC : Inport  SampleTime=Ts
  __UniqueOutportName__1__ : Outport
  wires:
  DC/1 -> __UniqueOutportName__1__/1

== system BLDCmotor_FOC_R2017b_fixdt_backup/PWM_gates/PWM_generator2/__OutputSSForSFun__ ==
  __UniqueInportName__1__ : Inport
  PWM : Outport
  wires:
  __UniqueInportName__1__/1 -> PWM/1

== system BLDCmotor_FOC_R2017b_fixdt_backup/PWM_gates/PWM_generator3/__InputSSForSFun__ ==
  DC : Inport  SampleTime=Ts
  __UniqueOutportName__1__ : Outport
  wires:
  DC/1 -> __UniqueOutportName__1__/1

== system BLDCmotor_FOC_R2017b_fixdt_backup/PWM_gates/PWM_generator3/__OutputSSForSFun__ ==
  __UniqueInportName__1__ : Inport
  PWM : Outport
  wires:
  __UniqueInportName__1__/1 -> PWM/1

== system BLDCmotor_FOC_R2017b_fixdt_backup/PWM_gates/PWM_generator4/__InputSSForSFun__ ==
  DC : Inport  SampleTime=Ts
  __UniqueOutportName__1__ : Outport
  wires:
  DC/1 -> __UniqueOutportName__1__/1

== system BLDCmotor_FOC_R2017b_fixdt_backup/PWM_gates/PWM_generator4/__OutputSSForSFun__ ==
  __UniqueInportName__1__ : Inport
  PWM : Outport
  wires:
  __UniqueInportName__1__/1 -> PWM/1

== system BLDCmotor_FOC_R2017b_fixdt_backup/PWM_gates/PWM_generator5/__InputSSForSFun__ ==
  DC : Inport  SampleTime=Ts
  __UniqueOutportName__1__ : Outport
  wires:
  DC/1 -> __UniqueOutportName__1__/1

== system BLDCmotor_FOC_R2017b_fixdt_backup/PWM_gates/PWM_generator5/__OutputSSForSFun__ ==
  __UniqueInportName__1__ : Inport
  PWM : Outport
  wires:
  __UniqueInportName__1__/1 -> PWM/1

== system BLDCmotor_FOC_R2017b_fixdt_backup/BLDC_controller/F01_Estimations/F01_04_Speed_Estimation/Raw_Motor_Speed_Estimation ==
  note: Speed calculations:
      | Speed_radps = (f_ctrl_Hz * Mechanical_angle_radps) / z_counter
      | cf_spd_coef = f_ctrl_Hz * Mechanical_angle_deg * pi/180 * 30/pi
      | Speed_radps = cf_spd_coef / z_counter
  note: Counter hold
  note: • In steady state, switch to 4 interval speed calculation for better accuracy.
      | • In transient, switch to 1 interval interval spped calculation for fast detection of the speed change.
  note: This switch is to manage when direction changes. In this case, the counter measures both the time to go and return (so twice the time) within the Hall change. However, the angle to stand-still is not known. As a work around just use the previous motor speed in absolute value.
  note: At stand-still the Hall sensor toggles if the motor is stoped at the edge of Hall change. This switch is to manage this situation and avoid unexpected behavior.
  z_dir : Inport
  z_dirPrev : Inport  Port=2
  z_counterRawPrev : Inport  Port=3
  n_motAbsPrev : Inport  Port=4
  Action Port : ActionPort  ActionType=then
  Abs2 : Abs  OutDataTypeStr=Inherit: Inherit via back propagation  RndMeth=Zero
  Constant4 : Constant  Value=0  OutDataTypeStr=Inherit: Inherit via back propagation
  Divide11 : Product  Inputs=**  RndMeth=Simplest  OutDataTypeStr=Inherit: Same as first input
  Divide13 : Product  Inputs=*/  OutDataTypeStr=fixdt(1,16,4)  RndMeth=Simplest
  Divide14 : Product  Inputs=*/  OutDataTypeStr=fixdt(1,16,4)  RndMeth=Simplest
  Logical Operator1 : Logic  AllPortsSameDT=off  OutDataTypeStr=boolean
  Relational Operator4 : RelationalOperator  Operator=~=  OutDataTypeStr=boolean  RndMeth=Simplest
  Sum13 : Sum  Inputs=++++  RndMeth=Simplest  InputSameDT=on  OutDataTypeStr=Inherit: Same as first input
  Sum7 : Sum  Inputs=+-  RndMeth=Simplest  InputSameDT=on  OutDataTypeStr=Inherit: Same as first input
  Switch1 : Switch  Tag=struct('comment',struct('text','','placement',1),'logdata',struct('maxnumvals',inf,'plotchannels',[],'loggingmode',3,'channels',1),'output',struct('variable','','description','','name','$S_$B','width',1,'address','','max',NaN,'min',NaN,'class','default','type','CONTINUOUS','scaling','','lsb',1,'offset',0,'arb',0,'freeze',1,'unit','','autoscalingmode',1,'lowerheadroom',1,'upperheadroom',1,'headroomunit','bit','keepdatatype',1,'checkmin',0,'checkmax',0,'castoutput',0,'show',0),'threshold',struct('variable','','description','','name','$S_$B_threshold','width',1,'address','','max',NaN,'min',NaN,'class','default','type','CONTINUOUS','scaling','','lsb',1,'offset',0,'arb',0,'freeze',1,'unit','','keepdatatype',1,'value','0','scalar',0,'criteria',3),'scalingvalid',0,'date',733087.49614628474,'inheritscaling',0)  Criteria=u2 ~= 0  InputSameDT=on
      settings: AttributesFormatString=threshold=%<threshold>\nCriteria : %<Criteria>
  Switch2 : Switch  Tag=struct('comment',struct('text','','placement',1),'logdata',struct('maxnumvals',inf,'plotchannels',[],'loggingmode',3,'channels',1),'output',struct('variable','','description','','name','$S_$B','width',1,'address','','max',NaN,'min',NaN,'class','default','type','CONTINUOUS','scaling','','lsb',1,'offset',0,'arb',0,'freeze',1,'unit','','autoscalingmode',1,'lowerheadroom',1,'upperheadroom',1,'headroomunit','bit','keepdatatype',1,'checkmin',0,'checkmax',0,'castoutput',0,'show',0),'threshold',struct('variable','','description','','name','$S_$B_threshold','width',1,'address','','max',NaN,'min',NaN,'class','default','type','CONTINUOUS','scaling','','lsb',1,'offset',0,'arb',0,'freeze',1,'unit','','keepdatatype',1,'value','0','scalar',0,'criteria',3),'scalingvalid',0,'date',733087.49614628474,'inheritscaling',0)  Criteria=u2 ~= 0  InputSameDT=on
      settings: AttributesFormatString=threshold=%<threshold>\nCriteria : %<Criteria>
  Switch3 : Switch  Tag=struct('comment',struct('text','','placement',1),'logdata',struct('maxnumvals',inf,'plotchannels',[],'loggingmode',3,'channels',1),'output',struct('variable','','description','','name','$S_$B','width',1,'address','','max',NaN,'min',NaN,'class','default','type','CONTINUOUS','scaling','','lsb',1,'offset',0,'arb',0,'freeze',1,'unit','','autoscalingmode',1,'lowerheadroom',1,'upperheadroom',1,'headroomunit','bit','keepdatatype',1,'checkmin',0,'checkmax',0,'castoutput',0,'show',0),'threshold',struct('variable','','description','','name','$S_$B_threshold','width',1,'address','','max',NaN,'min',NaN,'class','default','type','CONTINUOUS','scaling','','lsb',1,'offset',0,'arb',0,'freeze',1,'unit','','keepdatatype',1,'value','0','scalar',0,'criteria',3),'scalingvalid',0,'date',733087.49614628474,'inheritscaling',0)  Criteria=u2 ~= 0  InputSameDT=on
      settings: AttributesFormatString=threshold=%<threshold>\nCriteria : %<Criteria>
  UnitDelay{1..5} (5 alike) : UnitDelay  SampleTime=-1
      settings: AttributesFormatString=Ini=%<X0>
  cf_speedCoef : Constant  Value=cf_speedCoef  OutDataTypeStr=fixdt(0,16,0)
  dz_cntTrnsDet : Relay  OnSwitchValue=dz_cntTrnsDetHi  OffSwitchValue=dz_cntTrnsDetLo  OutDataTypeStr=boolean
  g_Ha : Gain  Gain=4  OutDataTypeStr=Inherit: Inherit via back propagation  RndMeth=Zero  ParamDataTypeStr=Inherit: Same as input
  z_counter : Outport  InitialOutput=z_maxCntRst
  dz_trnsDet : Outport  Port=2
  n_motRaw : Outport  Port=3
  wires:
  z_dir/1 -> [z_dir]
  z_dirPrev/1 -> [z_dirPrev]
  z_counterRawPrev/1 -> [z_counterRawPrev]
  [z_dir] -> Divide11/2
  UnitDelay3/1 -> UnitDelay2/1, Sum13/2
  UnitDelay5/1 -> UnitDelay3/1, Sum13/3
  [z_counter] -> UnitDelay5/1, Sum13/4
  [cf_speedCoef] -> g_Ha/1
  Sum13/1 -> Divide13/2
  g_Ha/1 -> Divide13/1
  [z_counter] -> Divide14/2
  [cf_speedCoef] -> Divide14/1
  UnitDelay4/1 -> Sum7/2
  [z_counter] -> UnitDelay4/1, Sum7/1
  Sum7/1 -> Abs2/1
  Abs2/1 -> dz_cntTrnsDet/1
  cf_speedCoef/1 -> [cf_speedCoef]
  UnitDelay2/1 -> Sum13/1
  [z_dir] -> Relational Operator4/1
  [z_dirPrev] -> Relational Operator4/2
  UnitDelay1/1 -> Logical Operator1/2
  Relational Operator4/1 -> UnitDelay1/1, Switch2/2, Logical Operator1/1
  Logical Operator1/1 -> Switch3/2
  Switch2/1 -> Switch3/3
  Constant4/1 -> Switch3/1
  Switch3/1 -> Divide11/1
  n_motAbsPrev/1 -> [n_motAbsPrev]
  [n_motAbsPrev] -> Switch2/1
  [z_counterRawPrev] -> z_counter/1, [z_counter]
  dz_cntTrnsDet/1 -> [dz_trnsDet], dz_trnsDet/1
  Divide13/1 -> Switch1/3
  Divide11/1 -> n_motRaw/1
  [dz_trnsDet] -> Switch1/2
  Switch1/1 -> Switch2/3
  Divide14/1 -> Switch1/1

== system BLDCmotor_FOC_R2017b_fixdt_backup/BLDC_controller/F03_Control_Mode_Manager/F03_03_Input_Target_Synthesis/Default_Control_Type ==
  r_inpTgt : Inport
  Action Port : ActionPort  ActionType=else
  r_inpTgtScaDft : Outport
  wires:
  r_inpTgt/1 -> r_inpTgtScaDft/1

== system BLDCmotor_FOC_R2017b_fixdt_backup/BLDC_controller/F03_Control_Mode_Manager/F03_03_Input_Target_Synthesis/Default_Mode ==
  r_inpTgtScaRaw : Inport
  Action Port : ActionPort  InitializeStates=reset  ActionType=else
  r_inpTgtScaDft : Outport
  wires:
  r_inpTgtScaRaw/1 -> r_inpTgtScaDft/1

== system BLDCmotor_FOC_R2017b_fixdt_backup/BLDC_controller/F03_Control_Mode_Manager/F03_03_Input_Target_Synthesis/FOC_Control_Type ==
  r_inpTgt : Inport
  z_ctrlModReq : Inport  Port=2
  Action Port : ActionPort  ActionType=then
  Divide1 : Product  Inputs=**  RndMeth=Simplest  OutDataTypeStr=Inherit: Same as first input
  Divide4 : Product  Inputs=*/  OutDataTypeStr=fixdt(0,16,12)  RndMeth=Simplest
  Mux : Mux
  Selector : Selector  IndexMode=Zero-based  InputPortWidth=4  IndexOptions=Index vector (port)  Indices=[1 3]  OutputSizes=1
  Vd_max : Constant  Value=Vd_max  OutDataTypeStr=fixdt(1,16,4)
  constant : Constant  Value=1000  OutDataTypeStr=Inherit: Inherit via back propagation
  constant1 : Constant  Value=0  OutDataTypeStr=Inherit: Inherit via back propagation
  i_max : Constant  Value=i_max  OutDataTypeStr=fixdt(1,16,4)
  n_max : Constant  Value=n_max  OutDataTypeStr=fixdt(1,16,4)
  r_inpTgtScaFOC : Outport
  wires:
  r_inpTgt/1 -> [r_inpTgt]
  [r_inpTgtScaFOC] -> r_inpTgtScaFOC/1
  z_ctrlModReq/1 -> [z_ctrlModReq]
  constant/1 -> Divide4/2
  Selector/1 -> Divide4/1
  constant1/1 -> Mux/1
  i_max/1 -> Mux/4
  Vd_max/1 -> Mux/2
  Mux/1 -> Selector/1
  n_max/1 -> Mux/3
  [z_ctrlModReq] -> Selector/2
  Divide4/1 -> Divide1/2
  Divide1/1 -> [r_inpTgtScaFOC]
  [r_inpTgt] -> Divide1/1
